simulink model "Battery_soc_simulation"  (R2025b)
settings: Solver=VariableStepAuto  StartTime=0.0  StopTime=10.0  RelTol=1e-3
settings Model: Creator=imman  LastModifiedBy=imman

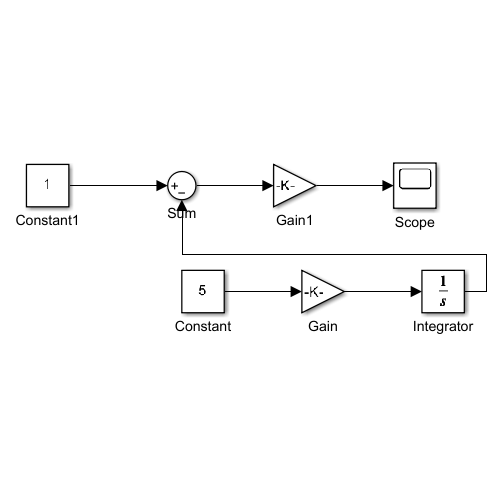
[thumbnail: Simulink's stored preview of the top-level diagram]
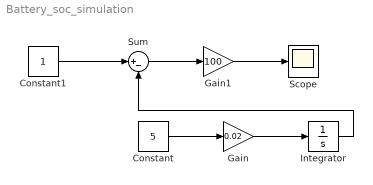
== system Battery_soc_simulation ==
  Constant : Constant  Value=5
  Constant1 : Constant
  Gain : Gain  Gain=0.02
  Gain1 : Gain  Gain=100
  Integrator : Integrator
  Scope : Scope
      settings: ActiveDisplayYMinimum=-42.172628153390093  ActiveDisplayYMaximum=172.37954513228655
  Sum : Sum  Inputs=|+-
  wires:
  Constant/1 -> Gain/1
  Gain/1 -> Integrator/1
  Constant1/1 -> Sum/1
  Integrator/1 -> Sum/2
  Sum/1 -> Gain1/1
  Gain1/1 -> Scope/1
